simulink model "LAB2_2_ssCT"  (R2025b)
settings: Solver=FixedStepAuto  StartTime=0.0  StopTime=10.0  FixedStep=0.0001  RelTol=1e-3
values from neighbouring files (symbols this model uses):
  Ao = -(1/Tm) - L    [LAB2_2_ssDT.m]
  Bo = [Km/(gbox.N*Tm), (-(1/Tm) - L)*L]    [LAB2_2_ssDT.m]
  Co = [0; 1]    [LAB2_2_ssDT.m]
  Do = [0, 1; 0, L]    [LAB2_2_ssDT.m]
  K = K2    [LAB2_2_ssDT.m]
  Ki = 0    [LAB2_2_ssDT.m]
  Nr = Nr2    [LAB2_2_ssDT.m]
undefined symbols (not defined in the file or in its folder): Beq, daq, drv, gbox, Jeq, mot, pulse2deg, rads2rpm, Req, Tausf
settings Model: Creator=ester  LastModifiedBy=ester

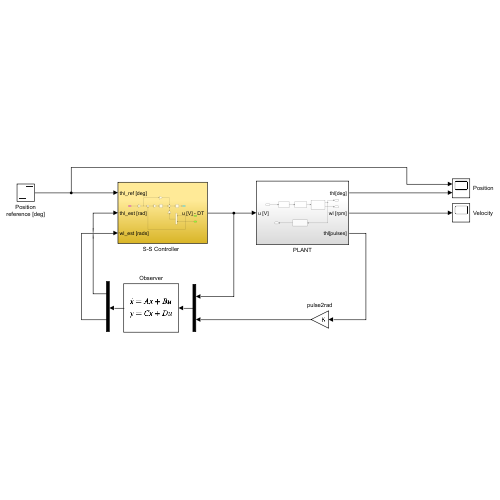
[thumbnail: Simulink's stored preview of the top-level diagram]
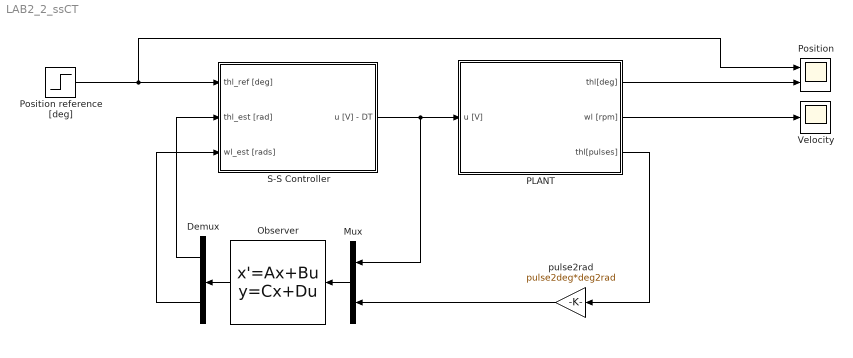
== system LAB2_2_ssCT ==
  Demux : Demux  Outputs=2
  Mux : Mux  Inputs=2
  Observer : StateSpace  A=Ao  B=Bo  C=Co  D=Do  InitialCondition=0
  PLANT : Subsystem
  Position : Scope  NumInputPorts=2
      settings: ActiveDisplayYMinimum=-7.4775977421854751  ActiveDisplayYMaximum=67.2983796796693
  Position reference [deg] : Step  Time=0  After=40  SampleTime=0  ZeroCross=off
  "S-S Controller  " : Subsystem
  Velocity : Scope
      settings: ActiveDisplayYMinimum=-1  ActiveDisplayYMaximum=1
  pulse2rad : Gain  Gain=pulse2deg*deg2rad
  wires:
  PLANT/1(thl[deg]) -> Position/2
  Position reference [deg]/1 -> "S-S Controller  "/1(thl_ref [deg]), Position/1
  "S-S Controller  "/1("u [V] - DT ") -> Mux/1, PLANT/1(u [V])
  PLANT/3(thl[pulses]) -> pulse2rad/1
  pulse2rad/1 -> Mux/2
  PLANT/2(wl [rpm]) -> Velocity/1
  Mux/1 -> Observer/1
  Observer/1 -> Demux/1
  Demux/1 -> "S-S Controller  "/2(thl_est [rad])
  Demux/2 -> "S-S Controller  "/3(wl_est [rads])

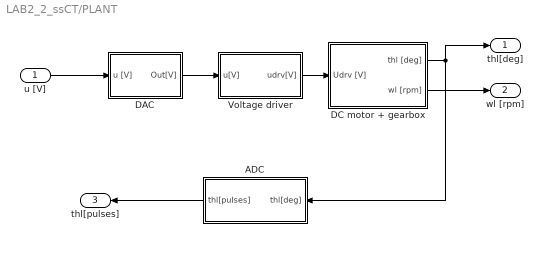
== system LAB2_2_ssCT/PLANT ==
  u [V] : Inport
  ADC : Subsystem  TreatAsAtomicUnit=on
  DAC : Subsystem  TreatAsAtomicUnit=on
  DC motor + gearbox : Subsystem
  Voltage driver : Subsystem  TreatAsAtomicUnit=on
  thl[deg] : Outport
  wl [rpm] : Outport  Port=2
  thl[pulses] : Outport  Port=3
  wires:
  DAC/1(Out[V]) -> Voltage driver/1(u[V])
  DC motor + gearbox/1(thl [deg]) -> thl[deg]/1, ADC/1(thl[deg])
  ADC/1(thl[pulses]) -> thl[pulses]/1
  u [V]/1 -> DAC/1(u [V])
  Voltage driver/1(udrv[V]) -> DC motor + gearbox/1(Udrv [V])
  DC motor + gearbox/2(wl [rpm]) -> wl [rpm]/1

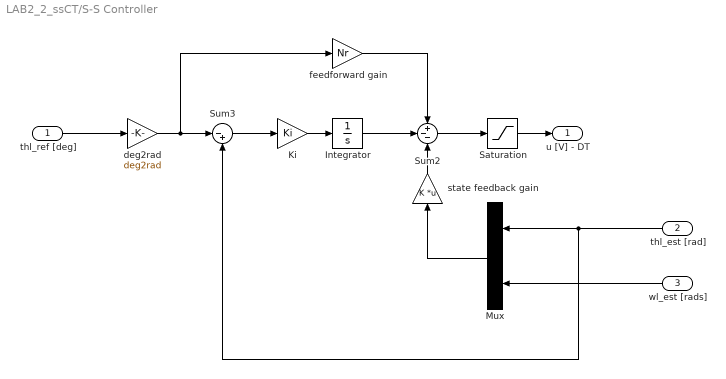
== system LAB2_2_ssCT/S-S Controller   ==
  thl_ref [deg] : Inport
  thl_est [rad] : Inport  Port=2
  wl_est [rads] : Inport  Port=3
  " feedforward gain" : Gain  Gain=Nr
  Integrator : Integrator
  Ki : Gain  Gain=Ki
  Mux : Mux  Inputs=2
  Saturation : Saturate  UpperLimit=10  LowerLimit=-10  ZeroCross=off
  Sum2 : Sum  Inputs=+--
  Sum3 : Sum  Inputs=|-+
  deg2rad : Gain  Gain=deg2rad
  state feedback gain : Gain  Gain=K  Multiplication=Matrix(K*u)
  "u [V] - DT " : Outport
  wires:
  wl_est [rads]/1 -> Mux/2
  thl_ref [deg]/1 -> deg2rad/1
  thl_est [rad]/1 -> Sum3/2, Mux/1
  " feedforward gain"/1 -> Sum2/1
  Integrator/1 -> Sum2/2
  Mux/1 -> state feedback gain/1
  Sum3/1 -> Ki/1
  state feedback gain/1 -> Sum2/3
  deg2rad/1 -> " feedforward gain"/1, Sum3/1
  Ki/1 -> Integrator/1
  Sum2/1 -> Saturation/1
  Saturation/1 -> "u [V] - DT "/1

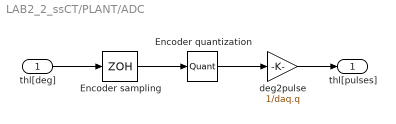
== system LAB2_2_ssCT/PLANT/ADC ==
  thl[deg] : Inport
  Encoder quantization : Quantizer  QuantizationInterval=daq.q
  Encoder sampling : ZeroOrderHold  SampleTime=daq.dac.Ts
  deg2pulse : Gain  Gain=1/daq.q
  thl[pulses] : Outport
  wires:
  Encoder quantization/1 -> deg2pulse/1
  thl[deg]/1 -> Encoder sampling/1
  Encoder sampling/1 -> Encoder quantization/1
  deg2pulse/1 -> thl[pulses]/1

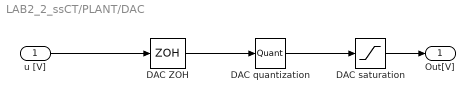
== system LAB2_2_ssCT/PLANT/DAC ==
  u [V] : Inport
  "DAC ZOH " : ZeroOrderHold  SampleTime=daq.dac.Ts
  DAC quantization : Quantizer  QuantizationInterval=daq.dac.q
  DAC saturation : Saturate  UpperLimit=daq.dac.fs  LowerLimit=-daq.dac.fs
  Out[V] : Outport
  wires:
  DAC quantization/1 -> DAC saturation/1
  u [V]/1 -> "DAC ZOH "/1
  "DAC ZOH "/1 -> DAC quantization/1
  DAC saturation/1 -> Out[V]/1

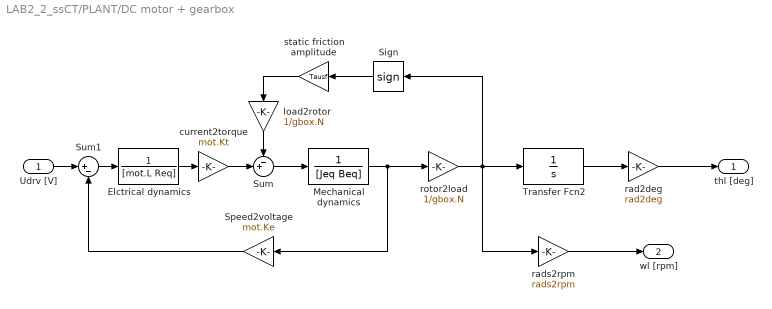
== system LAB2_2_ssCT/PLANT/DC motor + gearbox ==
  Udrv [V] : Inport
  Elctrical dynamics : TransferFcn  Denominator=[mot.L Req]
  Mechanical dynamics : TransferFcn  Denominator=[Jeq Beq]
  Sign : Signum  ZeroCross=off
  Speed2voltage : Gain  Gain=mot.Ke
  Sum : Sum  Inputs=-+|
  Sum1 : Sum  Inputs=|+-
  Transfer Fcn2 : TransferFcn  Denominator=[1 0]
  current2torque : Gain  Gain=mot.Kt
  load2rotor : Gain  Gain=1/gbox.N
  rad2deg : Gain  Gain=rad2deg
  rads2rpm : Gain  Gain=rads2rpm
  rotor2load : Gain  Gain=1/gbox.N
  static friction amplitude : Gain  Gain=Tausf
  thl [deg] : Outport
  wl [rpm] : Outport  Port=2
  wires:
  rotor2load/1 -> Sign/1, rads2rpm/1, Transfer Fcn2/1
  Sign/1 -> static friction amplitude/1
  rads2rpm/1 -> wl [rpm]/1
  Sum/1 -> Mechanical dynamics/1
  Udrv [V]/1 -> Sum1/1
  static friction amplitude/1 -> load2rotor/1
  load2rotor/1 -> Sum/1
  Transfer Fcn2/1 -> rad2deg/1
  current2torque/1 -> Sum/2
  Speed2voltage/1 -> Sum1/2
  Mechanical dynamics/1 -> Speed2voltage/1, rotor2load/1
  Elctrical dynamics/1 -> current2torque/1
  Sum1/1 -> Elctrical dynamics/1
  rad2deg/1 -> thl [deg]/1

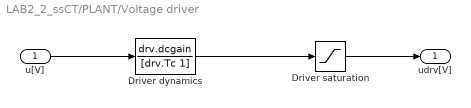
== system LAB2_2_ssCT/PLANT/Voltage driver ==
  u[V] : Inport
  Driver dynamics : TransferFcn  Numerator=drv.dcgain  Denominator=[drv.Tc 1]
  Driver saturation : Saturate  UpperLimit=drv.outmax  LowerLimit=-drv.outmax
  udrv[V] : Outport
  wires:
  Driver dynamics/1 -> Driver saturation/1
  u[V]/1 -> Driver dynamics/1
  Driver saturation/1 -> udrv[V]/1
